simulink model "ADAMS_ControlSystem_1"  (Simulink 8.3)
settings: Solver=FixedStepDiscrete  StartTime=0.0  StopTime=30  FixedStep=Ts  RelTol=1e-3
values from neighbouring files (symbols this model uses):
  K = (2*b*g)/(V^2)    (= 9.24143827911)    [startUp_conSys_bicycle_1_vR2014a.m]
  Rrw = .6482150285/2    (= 0.32410751425)    [startUp_conSys_bicycle_1_vR2014a.m]
  Ts = 1/100    (= 0.01)    [startUp_conSys_bicycle_1_vR2014a.m]
undefined symbols (not defined in the file): ADAMS_cwd, ADAMS_exec, ADAMS_host, ADAMS_init, ADAMS_inputs, ADAMS_outputs, ADAMS_prefix, ADAMS_static, ADAMS_sysdir
libraries: cstblocks x1
settings Model: Creator=baqumau  LastModifiedBy=baqumau
settings DataIOCC: SignalLoggingSaveFormat=Dataset
settings DebuggingCC: UnderspecifiedInitializationDetection=Simplified  StateNameClashWarn=none
settings GRTTargetCC: CombineOutputUpdateFcns=on  GRTInterface=off

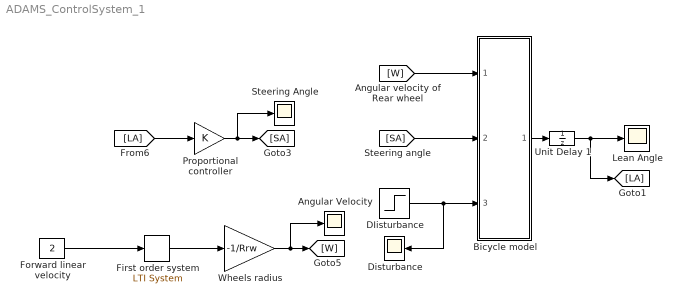
== system ADAMS_ControlSystem_1 ==
  Angular Velocity : Scope
      settings: SaveName=ScopeData3
  Bicycle model : Subsystem
  DIisturbance : Step  Time=10  After=5  SampleTime=Ts
  Disturbance : Scope
      settings: YMin=-3  YMax=8  SaveName=ScopeData2
  First order system : cstblocks/LTI System  sys=Fz  IC=[]
  Forward linear velocity : Constant  Value=2
  Lean Angle : Scope
  Proportional controller : Gain  Gain=K
  Steering Angle : Scope
  Unit Delay 1 : UnitDelay  SampleTime=Ts
  Wheels radius : Gain  Gain=-1/Rrw
  wires:
  [W] -> Bicycle model/1(Rear Wheel - Angular Velocity)
  DIisturbance/1 -> Disturbance/1, Bicycle model/3(Disturbance)
  [SA] -> Bicycle model/2(Steering Angle)
  Bicycle model/1(Lean Angle) -> Unit Delay 1/1
  Forward linear velocity/1 -> First order system/1
  Wheels radius/1 -> Angular Velocity/1, [W]
  [LA] -> Proportional controller/1
  Proportional controller/1 -> Steering Angle/1, [SA]
  First order system/1 -> Wheels radius/1
  Unit Delay 1/1 -> [LA], Lean Angle/1

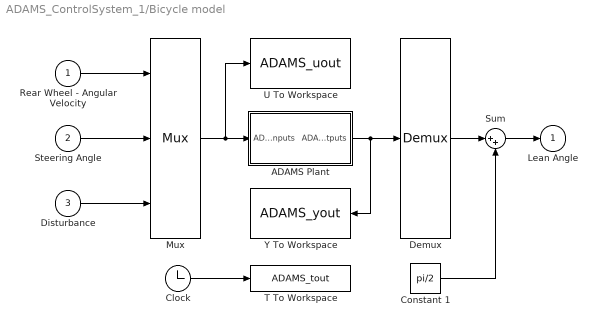
== system ADAMS_ControlSystem_1/Bicycle model ==
  Rear Wheel - Angular Velocity : Inport
  Steering Angle : Inport  Port=2
  Disturbance : Inport  Port=3
  ADAMS Plant : Subsystem  LoadFcn=|  InitFcn=clear mex  mask(Adams Plant){exevie=ADAMS_sysdir, nam_in=ADAMS_inputs, namout=ADAMS_outputs, nampre=ADAMS_prefix, outfil=ADAMS_prefix, exesol=ADAMS_exec, stat=ADAMS_static, inicmd=[ADAMS_init], exetyp=C++, comtyp=PIPE(DDE), workdir=ADAMS_cwd, ada_host=ADAMS_host, modani=batch, modsim=discrete, dft=no, simulink_lead_cosim=yes, pin_interp_order=0, pout_extrap_order=0, pin_extrap_order=0, pout_interp_order=0, dt_out=Ts, o_rate=1, more=off}
      | %check based on dialog box setting for when setting by popup menu                                             
      | if exist('ADAMS_solver_type')                                                                                 
      |   if strcmp(ADAMS_solver_type,'C++')                                                                          
      |     set_param(gcb,'exetyp','C++');                                                                            
      |   else                                                                                                        
      |     set_param(gcb,'exetyp','Fortran');                                                                        
      |   end                                                                                                         
      | else                                                                                                          
      |   set_param(gcb,'exetyp','C++');                                                                              
      | end                                                                                                           
      | %set the mode if using acar_solver                                                                            
      | %REQUIRED HERE BECAUSE BELOW CAUSES MDLTERMINATE TO BE CALLED 2 TIMES IN MIDDLE OF SIMULATION WHEN SET IN MASK
      |                                                                                                               
      | %enable the direct feedthrough, sim mode, anim mode parameters by default                                     
      |                                                                                                               
      | if exist('set_some_params_states')                                                                            
      |                                                                                                               
      |   set_some_params_states({'dft','modsim','modani'},{'on','on','on'},'MaskEnables',gcb)                        
      |   %turn on direct feedthrough option                                                                          
      |   set_some_params_states({'dft'},{'on'},'MaskVisibilities',gcb)                                               
      |                                                                                                               
      |  end                                                                                                          
      |                                                                                                               
      |                                                                                                               
      | if exist('ADAMS_exec')                                                                                        
      |   if and(strcmp(get_param(gcb,'exesol'),'ADAMS_exec'),strcmp(ADAMS_exec,'acar_solver'))                       
      |     %set the sim mode to discrete -- only supported mode                                                      
      |     set_param(gcb,'modsim','discrete')                                                                        
      |      %turn off direct feedthrough option                                                                      
      |      set_some_params_states({'dft'},{'off'},'MaskVisibilities',gcb)                                           
      |     %set the animation mode to batch -- only supported mode                                                   
      |     set_param(gcb,'modani','batch')                                                                           
      |     %disable the direct feedthrough, sim mode, anim mode parameters                                           
      |     set_some_params_states({'modsim','modani'},{'off','off'},'MaskEnables',gcb)                               
      |   end                                                                                                         
      | end
      mask prompts: exevie "Adams install directory"; nam_in "Adams/View input names"; namout "Adams/View output names"; nampre "Adams model file prefix"; outfil "Output files prefix (opt.: if blank - no output)"; exesol "User executable (opt.: if blank - use standard)"; stat "Initial static simulation flag"; inicmd "Initialization commands"; exetyp "Adams/Solver type"; comtyp "Interprocess option"; workdir "Adams working directory"; ada_host "Adams host"; modani "Animation mode"; modsim "Simulation mode"; dft "Direct feedthrough"; simulink_lead_cosim "Discrete Computational Order - Simulink Leads Adams"; pin_interp_order "Plant input interpolation order"; pout_extrap_order "Plant output extrapolation order"; pin_extrap_order "Plant input extrapolation order"; pout_interp_order "Plant output interpolation order"; dt_out "Communication interval"; o_rate "Number of communications per output step"; more "More parameters"
      mask help: Simulate any Adams plant model either in Adams/Solver form (.adm file) or in Adams/View form (.cmd file)
      settings: OpenFcn=|
      | open_system(gcb,'mask')
      | if not(exist('set_some_params_states'))
      | 
      | warning('The script "set_some_params_states.m" cannot be found in the MATLAB PATH.  Cannot update the ADAMS Plant S-Function parameters.')
      | 
      | warning('Recommended action(optional):  run the Adams/Controls .m file first to help choose the correct settings in the Adams S-Function block.')
      | 
      | end
      mask Help:
      | <html>
      | This S-Function represents the non-linear Adams Plant with the inputs sent to the Adams model <br>
      |  and the outputs generated by the Adams model.  See the Adams/Controls documentation for more <br>
      | information.  This plant uses the following variables:<br>
      | <br>
      | <b>ADAMS_sysdir  :</b> Adams installation directory<br>
      | <b>ADAMS_inputs  :</b> Input variables View names vector<br>
      | <b>ADAMS_outputs :</b> Outputs variables View names vector<br>
      | <b>ADAMS_prefix  : </b>ADAMS model files prefix (.adm, .cmd); also doubles as output files prefix<br>
      | <b>ADAMS_exec :</b> Adams/Solver user library or keyword (e.g., acar_solver)<br>
      | <b>ADAMS_static :</b> yes|no - initial static before Co-simulation(discrete)/Function Evaluation(continuous)<br>
      | <b>ADAMS_init :</b>Initialization commands (i.e., Adams/View or Solver commands, depending on setting for Animation mode)<br>
      | <b>ADAMS_cwd : </b> Current working directory (for TCP/IP)<br>
      | <b>ADAMS_host : </b>Name of Adams server host (for TCP/IP)<br>
      | <b>ADAMS_mode :</b> Linear or non-linear (i.e., co-sim, function eval)<br>
      | <b>ADAMS_solver_type :</b>Fortran or C++ (used to set popup menu when first loaded) <br>
      | 
      | 
      | <br>
      | The following settings can be chosen:<br>
      | <br>
      | <b>Adams/Solver type:</b>  Fortran or C++ (will also set ADAMS_solver_type)<br>
      | <b>Interprocess option:</b> Pipe(DDE) or TCP/IP; TCP/IP can allow different machines run Adams and MATLAB<br>
      | <b>Animation mode:</b> batch (Solver, uses .adm) or interactive (View, uses .cmd)<br>
      | <b>Simulation mode:</b> discrete (Co-simulation) or continuous (Function Evaluation)<br>
      | <b>Discrete Computational Order - Simulink Lead Adams:</b> for discrete mode, chooses if Simulink leads the integration (yes) or lags (no);<br> if set to "no", can remove algebraic loop<br>
      | <b>Plant input interpolation order:</b> 0 = zero-order hold; 1 = linear (discrete mode only, where Simulink leads)<br>
      | <b>Plant output extrapolation order:</b> 0 = zero-order hold;1 = linear(discrete mode only, where Simulink leads)<br>
      | <b>Plant input extrapolation order:</b> 0 = zero-order hold; 1 = linear (discrete mode only, where Adams leads)<br>
      | <b>Plant output interpolation order:</b> 0 = zero-order hold;1 = linear(discrete mode only, where Adams leads)<br>
      | <b>Direct feedthrough:</b> yes|no - yes = Input directly effect output(continuous mode-only)<br>
      | <b>Communication interval:</b> Time step at which Co-simulation exchange information (e.g.,0.005); also controls <br>output for continuous mode (Function Evaluation)<br>
      | <b>Number of communications per output step: </b>Sets Adams output rate (.res, .req, .gra) integer value (default: 1)<br>
      | </html>
      mask Callback exesol:
      | if exist('set_some_params_states')
      | %enable the direct feedthrough, sim mode, anim mode parameters
      | set_some_params_states({'dft','modsim','modani'},{'on','on','on'},'MaskEnables',gcb)
      | %turn on direct feedthrough option
      | set_some_params_states({'dft'},{'on'},'MaskVisibilities',gcb)
      | end
      | 
      | if exist('ADAMS_exec')
      |   if and(strcmp(get_param(gcb,'exesol'),'ADAMS_exec'),strcmp(ADAMS_exec,'acar_solver'))
      |     %set the sim mode to discrete -- only supported mode
      |     %REMOVED:  BELOW CAUSES MDLTERMINATE TO BE CALLED 2 TIMES IN MIDDLE OF SIMULATION
      |     %Now in LoadFcn callback
      |     %set_param(gcb,'modsim','discrete')
      |      %turn off direct feedthrough option
      |     set_some_params_states({'dft'},{'off'},'MaskVisibilities',gcb)
      |     %set the animation mode to batch -- only supported mode
      |     %REMOVED:  BELOW CAUSES MDLTERMINATE TO BE CALLED 2 TIMES IN MIDDLE OF SIMULATION
      |     %Now in LoadFcn callback
      |     %set_param(gcb,'modani','batch')
      |     %disable the direct feedthrough, sim mode, anim mode parameters
      |     set_some_params_states({'modsim','modani'},{'off','off'},'MaskEnables',gcb)
      |   end
      | end
      mask TypeOptions exetyp: Fortran | C++
      mask Callback exetyp:
      | if strcmp(get_param(gcb,'exetyp'),'C++')
      |     ADAMS_solver_type='C++';
      | else
      |     ADAMS_solver_type='Fortran';
      | end
      mask TypeOptions comtyp: PIPE(DDE) | TCP/IP
      mask Callback comtyp:
      | if exist('set_some_params_states')
      | if strcmp(get_param(gcb,'comtyp'),'PIPE(DDE)')
      |     %turn off cwd, host options
      |     set_some_params_states({'ada_host','workdir'},{'off','off'},'MaskVisibilities',gcb)
      | else%if strcmp(get_param(gcb,'modsim'),'TCP/IP')
      |     %turn on cwd, host options
      |     set_some_params_states({'ada_host','workdir'},{'on','on'},'MaskVisibilities',gcb)
      | end
      | end
      mask TypeOptions modani: batch | interactive
      mask TypeOptions modsim: discrete | continuous
      mask Callback modsim:
      | if exist('set_some_params_states')
      | if strcmp(get_param(gcb,'modsim'),'discrete')
      |      %turn off direct feedthrough option
      |     set_some_params_states({'dft'},{'off'},'MaskVisibilities',gcb)
      |     %turn on discrete co-sim type if want to see more
      |     if strcmp(get_param(gcb,'more'),'on')
      |         set_some_params_states({'simulink_lead_cosim'},{'on'},'MaskVisibilities',gcb)
      |     end
      |     if strcmp(get_param(gcb,'simulink_lead_cosim'),'yes')
      |         %turn on interpolation/extrapolation options
      |         set_some_params_states({'pin_interp_order','pout_extrap_order',},{'on','on'},'MaskVisibilities',gcb)
      |     else
      |         set_some_params_states({'pin_extrap_order','pout_interp_order'},{'on','on'},'MaskVisibilities',gcb)
      |     end
      | else%if strcmp(get_param(gcb,'modsim'),'continuous')
      |      %turn off direct feedthrough option
      |     set_some_params_states({'dft'},{'on'},'MaskVisibilities',gcb)
      |     %turn off interpolation/extrapolation options
      |     set_some_params_states({'pin_interp_order','pout_extrap_order','pin_extrap_order','pout_interp_order','simulink_lead_cosim'},{'off','off','off','off','off'},'MaskVisibilities',gcb)
      | end
      | end
      mask TypeOptions dft: no | yes
      mask TypeOptions simulink_lead_cosim: yes | no
      mask Callback simulink_lead_cosim:
      | if exist('set_some_params_states')
      | if (strcmp(get_param(gcb,'simulink_lead_cosim'),'yes') && strcmp(get_param(gcb,'modsim'),'discrete'))
      |      %turn off unused interpolate/extrapolate options
      |     set_some_params_states({'pin_extrap_order','pout_interp_order'},{'off','off'},'MaskVisibilities',gcb)
      |     %turn on used interpolate/extrapolate options
      |     set_some_params_states({'pin_interp_order','pout_extrap_order'},{'on','on'},'MaskVisibilities',gcb)
      | elseif (strcmp(get_param(gcb,'simulink_lead_cosim'),'no') && strcmp(get_param(gcb,'modsim'),'discrete'))
      |     %turn on used interpolate/extrapolate options
      |     set_some_params_states({'pin_extrap_order','pout_interp_order'},{'on','on'},'MaskVisibilities',gcb)
      |      %turn off unused interpolate/extrapolate options
      |     set_some_params_states({'pin_interp_order','pout_extrap_order'},{'off','off'},'MaskVisibilities',gcb)
      | end
      | end
      mask TypeOptions pin_interp_order: 0 | 1
      mask TypeOptions pout_extrap_order: 0 | 1
      mask TypeOptions pin_extrap_order: 0 | 1
      mask TypeOptions pout_interp_order: 0 | 1
      mask Callback more:
      | if exist('set_some_params_states')
      | if (strcmp(get_param(gcb,'more'),'on'))
      |      %turn on infrequently used options
      |     set_some_params_states({'exevie','nam_in','namout','exesol','stat','inicmd'},{'on','on','on','on','on','on'},'MaskVisibilities',gcb)
      |     if strcmp(get_param(gcb,'modsim'),'discrete')
      |         set_some_params_states({'simulink_lead_cosim'},{'on'},'MaskVisibilities',gcb)
      |     end
      | elseif (strcmp(get_param(gcb,'more'),'off'))
      |     %turn off infrequently used options
      |     set_some_params_states({'exevie','nam_in','namout','exesol','stat','inicmd'},{'off','off','off','off','off','off'},'MaskVisibilities',gcb)
      |     if strcmp(get_param(gcb,'modsim'),'discrete')
      |         set_some_params_states({'simulink_lead_cosim'},{'off'},'MaskVisibilities',gcb)
      |     end
      | end
      | end
      mask Display: disp( 'MSC Software' )
  Clock : Clock
  Constant 1 : Constant  Value=pi/2  SampleTime=Ts
  Demux : Demux  Outputs=1
  Mux : Mux  Inputs=3
  Sum : Sum  Inputs=|++
  T To Workspace : ToWorkspace  VariableName=ADAMS_tout
      settings: MaxDataPoints=100000
  U To Workspace : ToWorkspace  VariableName=ADAMS_uout
      settings: MaxDataPoints=100000
  Y To Workspace : ToWorkspace  VariableName=ADAMS_yout
      settings: MaxDataPoints=100000
  Lean Angle : Outport
  wires:
  Disturbance/1 -> Mux/3
  Steering Angle/1 -> Mux/2
  Rear Wheel - Angular Velocity/1 -> Mux/1
  ADAMS Plant/1(ADAMS outputs) -> Y To Workspace/1, Demux/1
  Mux/1 -> U To Workspace/1, ADAMS Plant/1(ADAMS inputs)
  Clock/1 -> T To Workspace/1
  Demux/1 -> Sum/1
  Sum/1 -> Lean Angle/1
  Constant 1/1 -> Sum/2

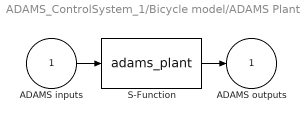
== system ADAMS_ControlSystem_1/Bicycle model/ADAMS Plant ==
  ADAMS inputs : Inport
  S-Function : S-Function  StopFcn=clear mex  FunctionName=adams_plant  Parameters=exevie,exesol,stat,outfil,nampre,o_rate,nam_in,namout,dft,modsim,modani,dt_out,inicmd,exetyp,comtyp,ada_host, workdir,pin_interp_order,pout_extrap_order,pin_extrap_order,pout_interp_order,simulink_lead_cosim  EnableBusSupport=off
  ADAMS outputs : Outport  InitialOutput=0
  wires:
  S-Function/1 -> ADAMS outputs/1
  ADAMS inputs/1 -> S-Function/1
